simulink model "PID_Drone_Controller_Simulink"  (R2021b)
settings: Solver=VariableStepAuto  StartTime=0.0  StopTime=200  FixedStep=0.001  MaxStep=0.4  RelTol=1e-3
libraries: slpidlib x1
settings Model: Creator=Wajih  LastModifiedBy=HP
settings SolverCC: ZeroCrossAlgorithm=Adaptive

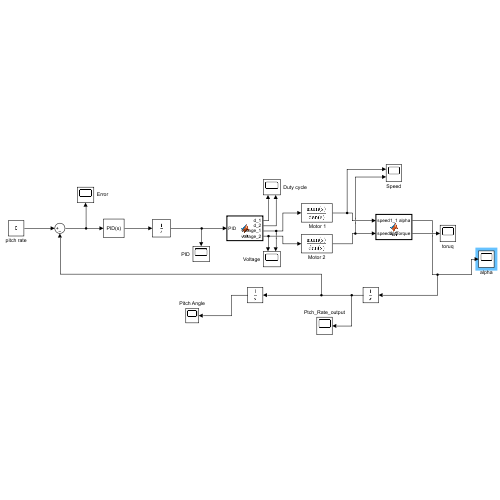
[thumbnail: Simulink's stored preview of the top-level diagram]
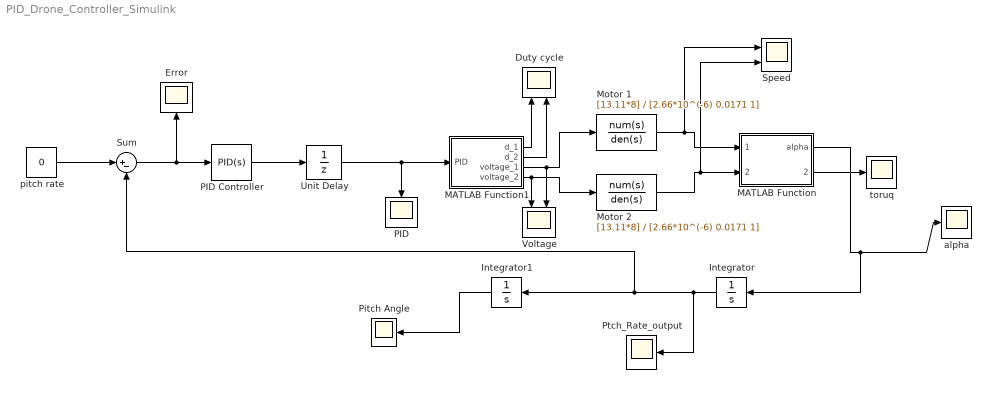
== system PID_Drone_Controller_Simulink ==
  " Motor 1" : TransferFcn  Numerator=[13.11*8]  Denominator=[2.66*10^(-6) 0.0171 1]
  Duty cycle : Scope  NumInputPorts=2
  Error : Scope
  Integrator : Integrator
  Integrator1 : Integrator
  MATLAB Function : MATLAB Function  TreatAsAtomicUnit=on
  MATLAB Function1 : MATLAB Function  TreatAsAtomicUnit=on
  Motor 2 : TransferFcn  Numerator=[13.11*8]  Denominator=[2.66*10^(-6) 0.0171 1]
  PID : Scope
  PID Controller : slpidlib/PID Controller  Controller=PID  Form=Parallel  TimeDomain=Continuous-time  UseExternalTs=off  SampleTime=-1  IntegratorMethod=Forward Euler  FilterMethod=Forward Euler  ControllerParametersSource=internal  P=7.5  I=0.2  D=1.5  UseFilter=on  N=1  TunerSelectOption=Transfer Function Based (PID Tuner App)  InitialConditionSource=internal  InitialConditionForIntegrator=0  InitialConditionForFilter=0  DifferentiatorICPrevScaledInput=0  ExternalReset=none  TrackingMode=off  Kt=1  LimitOutput=off  SatLimitsSource=internal  UpperSaturationLimit=inf  LowerSaturationLimit=-inf  LinearizeAsGain=on  AntiWindupMode=none  Kb=1  POutMin=[]  POutMax=[]  IOutMin=[]  IOutMax=[]  DOutMin=[]  DOutMax=[]  NOutMin=[]  NOutMax=[]  SumOutMin=[]  SumOutMax=[]  SaturationOutMin=[]  SaturationOutMax=[]  PParamMin=[]  PParamMax=[]  IParamMin=[]  IParamMax=[]  DParamMin=[]  DParamMax=[]  NParamMin=[]  NParamMax=[]  KbParamMin=[]  KbParamMax=[]  KtParamMin=[]  KtParamMax=[]  KbOutMin=[]  KbOutMax=[]  KtOutMin=[]  KtOutMax=[]  IntegratorOutMin=[]  IntegratorOutMax=[]  FilterOutMin=[]  FilterOutMax=[]  SumI1OutMin=[]  SumI1OutMax=[]  SumI2OutMin=[]  SumI2OutMax=[]  SumI3OutMin=[]  SumI3OutMax=[]  SumI4OutMin=[]  SumI4OutMax=[]  SumDOutMin=[]  SumDOutMax=[]  DifferentiatorOutMin=[]  DifferentiatorOutMax=[]  FilterDiffOutCoefMin=[]  FilterDiffOutCoefMax=[]  ReciprocalOutMin=[]  ReciprocalOutMax=[]  SumDenOutMin=[]  SumDenOutMax=[]  SumNumOutMin=[]  SumNumOutMax=[]  DivideOutMin=[]  DivideOutMax=[]  UdiffTsProdOutMin=[]  UdiffTsProdOutMax=[]  NTsProdOutMin=[]  NTsProdOutMax=[]  UintegralTsProdOutMin=[]  UintegralTsProdOutMax=[]  UngainTsProdOutMin=[]  UngainTsProdOutMax=[]  IntegratorContinuousStateAttributes=''  IntegratorStateMustResolveToSignalObject=off  IntegratorRTWStateStorageClass=Auto  FilterContinuousStateAttributes=''  FilterStateMustResolveToSignalObject=off  FilterRTWStateStorageClass=Auto  ParallelPVariant=InternalParameters  IdealPVariant=Disabled  IVariant=InternalParameters  DVariant=InternalParameters  IntegratorVariant=Continuous  SatVariant=Disabled  AWVariant=Passthrough  PCopyVariant=Disabled  TRVariant=Disabled  FdbkBlocksVariant=Forward  IdealPFdbkVariant=Disabled  SatFdbkVariant=Disabled  DerivativeFilterVariant=ContFilter  NVariant=InternalParameters  NCopyVariant=Disabled  FilterICVariant=InternalICsFilter  IntegratorICVariant=InternalICs  ExternalResetVariant=Disabled  TRSumVariant=Passthrough  SumFdbkVariant=Disabled  SumVariant=Sum_PID  TsampFilterVariant=InternalTs  TsampNgainVariant=Passthrough  TsampIntegralVariant=Passthrough  ExternalSaturationOutDataTypeStr=Inherit: Same as second input
  Pitch Angle : Scope
  Ptch_Rate_output : Scope
  Speed : Scope  NumInputPorts=2
  Sum : Sum  Inputs=|+-
  Unit Delay : UnitDelay  InitialCondition=100  SampleTime=-1  HasFrameUpgradeWarning=on
  Voltage : Scope  NumInputPorts=2
  alpha : Scope
  pitch rate : Constant  Value=0
  toruq : Scope
  wires:
  " Motor 1"/1 -> Speed/1, MATLAB Function/1(speed1_1)
  Motor 2/1 -> Speed/2, MATLAB Function/2(speed2_1)
  pitch rate/1 -> Sum/1
  MATLAB Function1/4(voltage_2) -> Voltage/1, Motor 2/1
  MATLAB Function1/1(d_1) -> Duty cycle/1
  MATLAB Function1/2(d_2) -> Duty cycle/2
  MATLAB Function1/3(voltage_1) -> Voltage/2, " Motor 1"/1
  MATLAB Function/2(netTorque) -> toruq/1
  MATLAB Function/1(alpha) -> Integrator/1, alpha/1
  Sum/1 -> PID Controller/1, Error/1
  Integrator/1 -> Ptch_Rate_output/1, Integrator1/1, Sum/2
  PID Controller/1 -> Unit Delay/1
  Unit Delay/1 -> PID/1, MATLAB Function1/1(PID)
  Integrator1/1 -> Pitch Angle/1

== matlab function PID_Drone_Controller_Simulink/MATLAB Function1 ==
  data: PID input; d_1 output; d_2 output; voltage_1 output; voltage_2 output
function [d_1,d_2,voltage_1,voltage_2] = fcn(PID)
throttle = 1300;
vmax = 4.2*3;
if(PID < -1000)

  PID=-1000;
end
if(PID > 1000)

  PID=1000;
end

pwmLeft = throttle - PID;
pwmRight = throttle + PID;

if(pwmRight < 1000)

  pwmRight= 1000;
end
if(pwmRight > 2000)

  pwmRight=2000;
end

if(pwmLeft < 1000)

  pwmLeft= 1000;
end
if(pwmLeft > 2000)

  pwmLeft=2000;
end
d_1 = pwmLeft/2000*100;
voltage_1 = d_1/100*vmax;
d_2 = pwmRight/2000*100;
voltage_2 = d_2/100*vmax;

== matlab function PID_Drone_Controller_Simulink/MATLAB Function ==
  data: speed1_1 input; alpha output; speed2_1 input; netTorque output
function [alpha,netTorque] = fcn(speed1_1, speed2_1)
    speed1 = speed1_1*(60/(2*pi));
    speed2 = speed2_1*(60/(2*pi));
    
    L=0.635;
    M = 0.15;
    thrust1 = 2.158242 + (0.03861053 - 2.158242)/(1 + (speed1/6670.543)^3.254664);
    thrust2 = 2.158242 + (0.03861053 - 2.158242)/(1 + (speed2/6670.543)^3.254664);
    torque1=thrust1*L/2;
    torque2=thrust2*L/2;
    netTorque = torque2 - torque1;
    MOI=(1/12)*M*L^2;
    alpha = netTorque/MOI;
end
